simulink model "RLS_Self_maglev"  (R2023b)
settings: Solver=VariableStepAuto  StartTime=0.0  StopTime=5  RelTol=1e-3
undefined symbols (not defined in the file or in its folder): A_ob, B_ob, C_ob, D_ob, x1_eq0, x2_eq0
settings Model: Creator=Simone Garatti  LastModifiedBy=lollo
settings SolverCC: AlgebraicLoopSolver=TrustRegion
settings DataIOCC: ReturnWorkspaceOutputs=off
settings DebuggingCC: UnconnectedInputMsg=warning  UnconnectedOutputMsg=warning  UnconnectedLineMsg=warning  ArithmeticOperatorsInVariantConditions=warning
settings ModelReferenceCC: EnableRefExpFcnMdlSchedulingChecks=on
settings SFSimCC: CustomCodeUndefinedFunction=UseInterfaceOnly

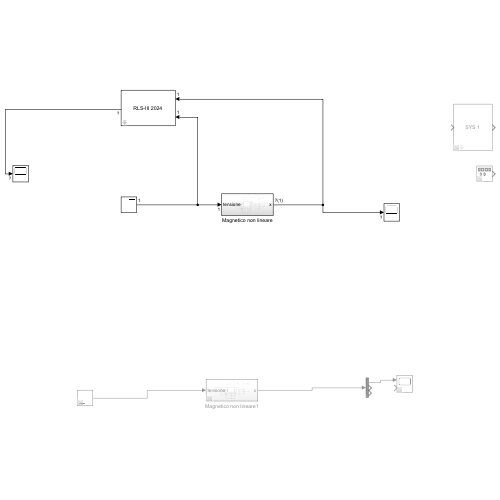
[thumbnail: Simulink's stored preview of the top-level diagram]
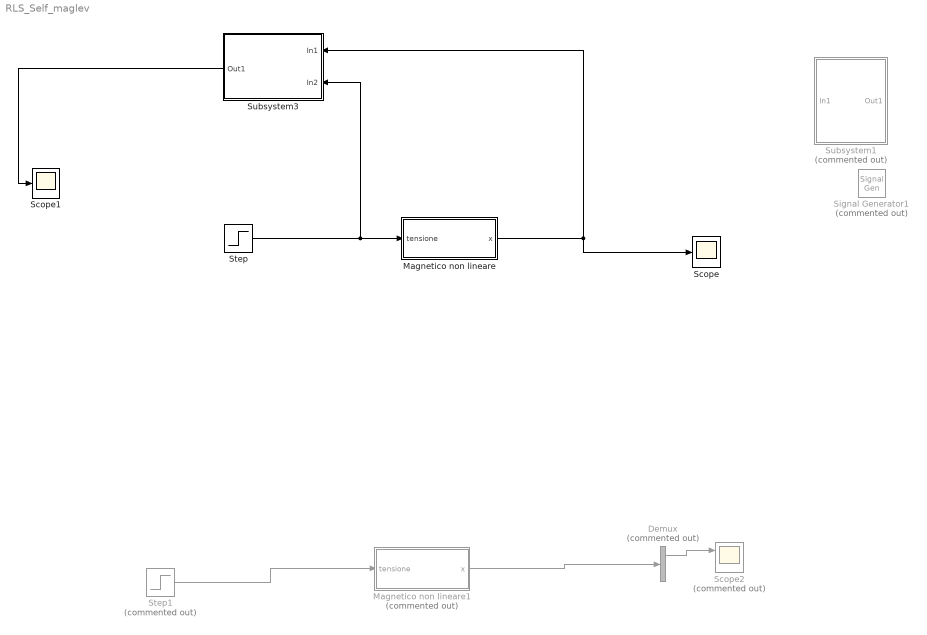
== system RLS_Self_maglev ==
  Demux : Demux  Commented=on  Outputs=3
  Magnetico non lineare : Subsystem
  Magnetico non lineare1 : Subsystem  Commented=on
  Scope : Scope
  Scope1 : Scope
  Scope2 : Scope  Commented=on  NumInputPorts=2
  Signal Generator1 : SignalGenerator  Commented=on  WaveForm=square  Frequency=0.01
  Step : Step  After=16  SampleTime=0
  Step1 : Step  Commented=on  After=20  SampleTime=0
  Subsystem1 : Subsystem  Commented=on  mask{yi=0, ui=0}
      mask prompts: yi "y(0)"; ui "u(0)"
      mask Display: disp('SYS 1')
  Subsystem3 : Subsystem  mask{th0=[2 3 2]', S0=eye(3)/100, ny=2, nu=0, d=1, mu=1}
      mask prompts: th0 "theta init"; S0 "S init"; d "u-y delay"; mu "forgetting factor"
      mask Display: disp('RLS-III 2024')
  wires:
  Step/1 -> Subsystem3/2(In2), Magnetico non lineare/1(tensione)
  Magnetico non lineare/1(x) -> Scope/1, Subsystem3/1(In1)
  Subsystem3/1(Out1) -> Scope1/1
  Step1/1 -> Magnetico non lineare1/1(tensione)
  Demux/1 -> Scope2/1
  Magnetico non lineare1/1(x) -> Demux/1

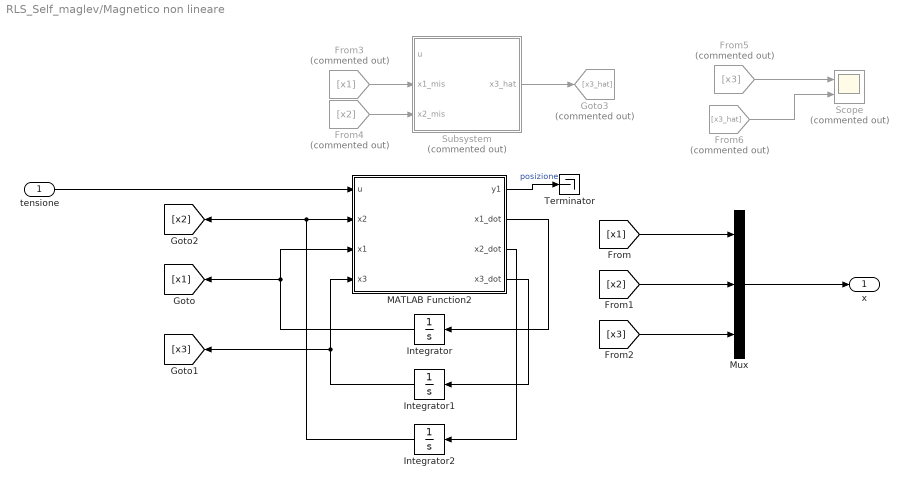
== system RLS_Self_maglev/Magnetico non lineare ==
  tensione : Inport
  From3 : From  Commented=on  GotoTag=x1
  From4 : From  Commented=on  GotoTag=x2
  From5 : From  Commented=on  GotoTag=x3
  From6 : From  Commented=on  GotoTag=x3_hat
  Goto3 : Goto  Commented=on  GotoTag=x3_hat
  Integrator : Integrator
  Integrator1 : Integrator
  Integrator2 : Integrator
  MATLAB Function2 : MATLAB Function  TreatAsAtomicUnit=on
  Mux : Mux  Inputs=3
  Scope : Scope  Commented=on  NumInputPorts=2
  Subsystem : Subsystem  Commented=on
  Terminator : Terminator
  x : Outport
  wires:
  tensione/1 -> MATLAB Function2/1(u)
  MATLAB Function2/2(x1_dot) -> Integrator/1
  Integrator/1 -> MATLAB Function2/3(x1), [x1]
  MATLAB Function2/4(x3_dot) -> Integrator1/1
  Integrator1/1 -> [x3], MATLAB Function2/4(x3)
  [x1] -> Mux/1
  [x2] -> Mux/2
  [x3] -> Mux/3
  Mux/1 -> x/1
  MATLAB Function2/3(x2_dot) -> Integrator2/1
  Integrator2/1 -> MATLAB Function2/2(x2), [x2]
  From3/1 -> Subsystem/2(x1_mis)
  From4/1 -> Subsystem/3(x2_mis)
  Subsystem/1(x3_hat) -> Goto3/1
  From6/1 -> Scope/2
  From5/1 -> Scope/1
  MATLAB Function2/1(y1) -> Terminator/1  "posizione"

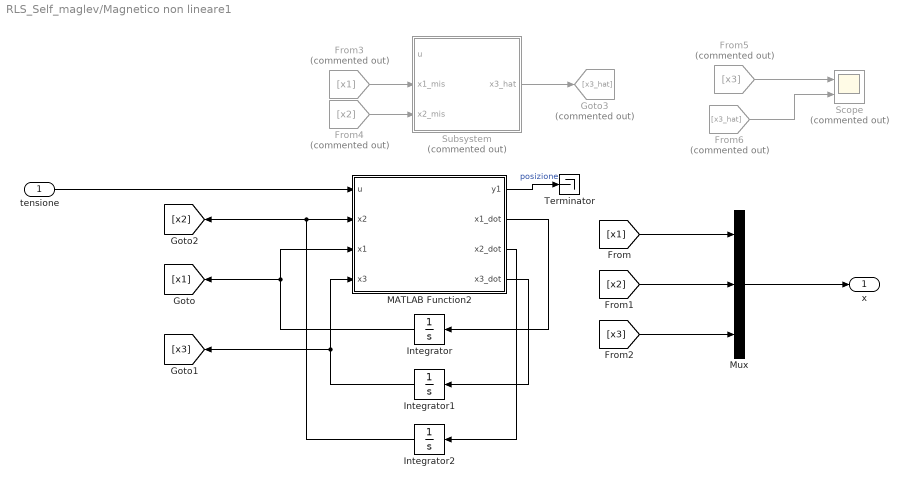
== system RLS_Self_maglev/Magnetico non lineare1 ==
  tensione : Inport
  From3 : From  Commented=on  GotoTag=x1
  From4 : From  Commented=on  GotoTag=x2
  From5 : From  Commented=on  GotoTag=x3
  From6 : From  Commented=on  GotoTag=x3_hat
  Goto3 : Goto  Commented=on  GotoTag=x3_hat
  Integrator : Integrator
  Integrator1 : Integrator
  Integrator2 : Integrator
  MATLAB Function2 : MATLAB Function  TreatAsAtomicUnit=on
  Mux : Mux  Inputs=3
  Scope : Scope  Commented=on  NumInputPorts=2
  Subsystem : Subsystem  Commented=on
  Terminator : Terminator
  x : Outport
  wires:
  tensione/1 -> MATLAB Function2/1(u)
  MATLAB Function2/2(x1_dot) -> Integrator/1
  Integrator/1 -> MATLAB Function2/3(x1), [x1]
  MATLAB Function2/4(x3_dot) -> Integrator1/1
  Integrator1/1 -> [x3], MATLAB Function2/4(x3)
  [x1] -> Mux/1
  [x2] -> Mux/2
  [x3] -> Mux/3
  Mux/1 -> x/1
  MATLAB Function2/3(x2_dot) -> Integrator2/1
  Integrator2/1 -> MATLAB Function2/2(x2), [x2]
  From3/1 -> Subsystem/2(x1_mis)
  From4/1 -> Subsystem/3(x2_mis)
  Subsystem/1(x3_hat) -> Goto3/1
  From6/1 -> Scope/2
  From5/1 -> Scope/1
  MATLAB Function2/1(y1) -> Terminator/1  "posizione"

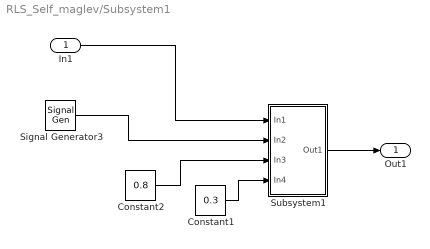
== system RLS_Self_maglev/Subsystem1 ==
  In1 : Inport
  Constant1 : Constant  Value=0.3
  Constant2 : Constant  Value=0.8
  Signal Generator3 : SignalGenerator  WaveForm=random  Amplitude=0.0  Frequency=0.01
  Subsystem1 : Subsystem  mask{y0=yi, u0=ui}
      mask prompts: y0 "y(0)"; u0 "u(0)"
      mask Display: disp('SYS')
  Out1 : Outport  VectorParamsAs1DForOutWhenUnconnected=off
  wires:
  Signal Generator3/1 -> Subsystem1/2(In2)
  Subsystem1/1(Out1) -> Out1/1
  Constant1/1 -> Subsystem1/4(In4)
  In1/1 -> Subsystem1/1(In1)
  Constant2/1 -> Subsystem1/3(In3)

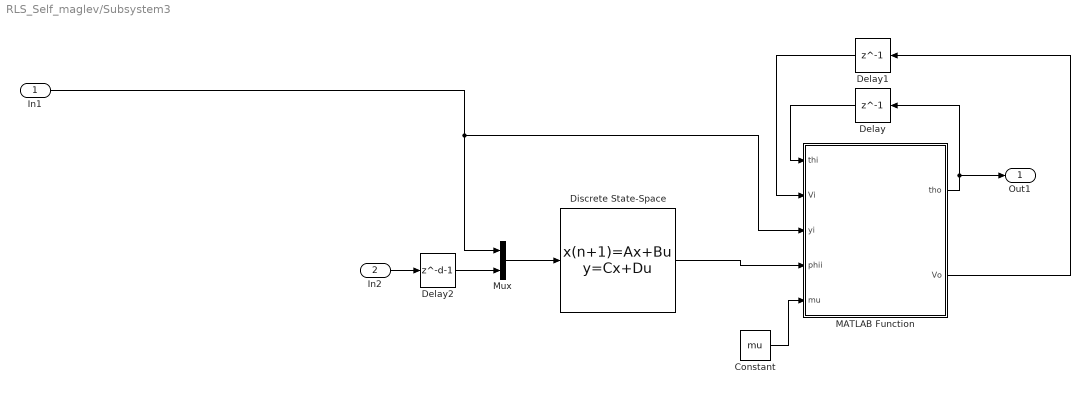
== system RLS_Self_maglev/Subsystem3 ==
  In1 : Inport
  In2 : Inport  Port=2
  Constant : Constant  Value=mu
  Delay : Delay  DelayLength=1  InitialCondition=th0
  Delay1 : Delay  DelayLength=1  InitialCondition=inv(S0)
  Delay2 : Delay  DelayLength=d-1  InitialCondition=0
  Discrete State-Space : DiscreteStateSpace  A=[ diag(ones(ny-1,1),-1) zeros(ny,nu+1); zeros(nu+1,ny) diag(ones(nu,1),-1) ]  B=[[1 0]; zeros(ny-1,2); [0 1]; zeros(nu,2)]  C=eye(ny+nu+1)  D=zeros(ny+nu+1,2)  SampleTime=-1
  MATLAB Function : MATLAB Function  TreatAsAtomicUnit=on
  Mux : Mux  Inputs=2
  Out1 : Outport  VectorParamsAs1DForOutWhenUnconnected=off
  wires:
  MATLAB Function/1(tho) -> Delay/1, Out1/1
  Delay/1 -> MATLAB Function/1(thi)
  MATLAB Function/2(Vo) -> Delay1/1
  Delay1/1 -> MATLAB Function/2(Vi)
  In1/1 -> Mux/1, MATLAB Function/3(yi)
  In2/1 -> Delay2/1
  Delay2/1 -> Mux/2
  Mux/1 -> Discrete State-Space/1
  Discrete State-Space/1 -> MATLAB Function/4(phii)
  Constant/1 -> MATLAB Function/5(mu)

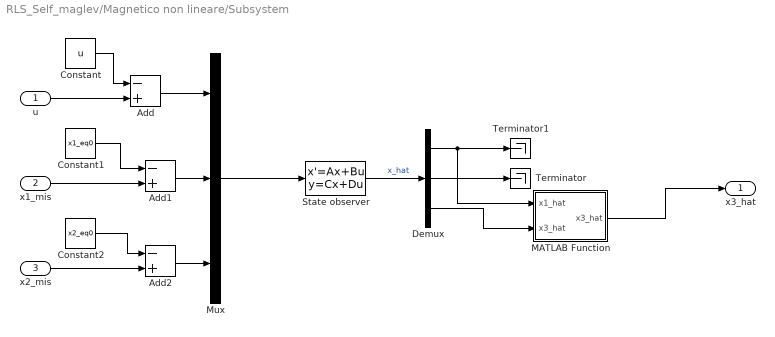
== system RLS_Self_maglev/Magnetico non lineare/Subsystem ==
  u : Inport
  x1_mis : Inport  Port=2
  x2_mis : Inport  Port=3
  Add : Sum  Inputs=-+
  Add1 : Sum  Inputs=-+
  Add2 : Sum  Inputs=-+
  Constant : Constant  Value=u
  Constant1 : Constant  Value=x1_eq0
  Constant2 : Constant  Value=x2_eq0
  Demux : Demux  Outputs=3
  MATLAB Function : MATLAB Function  TreatAsAtomicUnit=on
  Mux : Mux  Inputs=3
  State observer : StateSpace  A=A_ob  B=B_ob  C=C_ob  D=D_ob  InitialCondition=[0;0;0]  ParameterTunability=Unconstrained
  Terminator : Terminator
  Terminator1 : Terminator
  x3_hat : Outport
  wires:
  x1_mis/1 -> Add1/2
  u/1 -> Add/2
  Mux/1 -> State observer/1
  State observer/1 -> Demux/1  "x_hat"
  Demux/1 -> MATLAB Function/1(x1_hat), Terminator1/1
  Demux/2 -> Terminator/1
  Constant/1 -> Add/1
  Constant1/1 -> Add1/1
  Constant2/1 -> Add2/1
  x2_mis/1 -> Add2/2
  Add/1 -> Mux/1
  Add1/1 -> Mux/2
  Add2/1 -> Mux/3
  MATLAB Function/1(x3_hat) -> x3_hat/1
  Demux/3 -> MATLAB Function/2("x3_hat ")

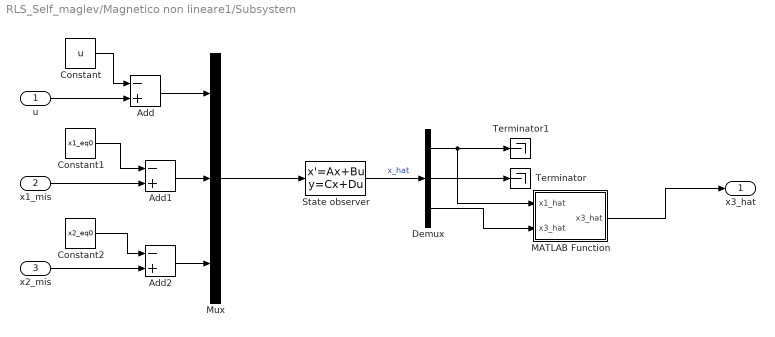
== system RLS_Self_maglev/Magnetico non lineare1/Subsystem ==
  u : Inport
  x1_mis : Inport  Port=2
  x2_mis : Inport  Port=3
  Add : Sum  Inputs=-+
  Add1 : Sum  Inputs=-+
  Add2 : Sum  Inputs=-+
  Constant : Constant  Value=u
  Constant1 : Constant  Value=x1_eq0
  Constant2 : Constant  Value=x2_eq0
  Demux : Demux  Outputs=3
  MATLAB Function : MATLAB Function  TreatAsAtomicUnit=on
  Mux : Mux  Inputs=3
  State observer : StateSpace  A=A_ob  B=B_ob  C=C_ob  D=D_ob  InitialCondition=[0;0;0]  ParameterTunability=Unconstrained
  Terminator : Terminator
  Terminator1 : Terminator
  x3_hat : Outport
  wires:
  x1_mis/1 -> Add1/2
  u/1 -> Add/2
  Mux/1 -> State observer/1
  State observer/1 -> Demux/1  "x_hat"
  Demux/1 -> MATLAB Function/1(x1_hat), Terminator1/1
  Demux/2 -> Terminator/1
  Constant/1 -> Add/1
  Constant1/1 -> Add1/1
  Constant2/1 -> Add2/1
  x2_mis/1 -> Add2/2
  Add/1 -> Mux/1
  Add1/1 -> Mux/2
  Add2/1 -> Mux/3
  MATLAB Function/1(x3_hat) -> x3_hat/1
  Demux/3 -> MATLAB Function/2("x3_hat ")

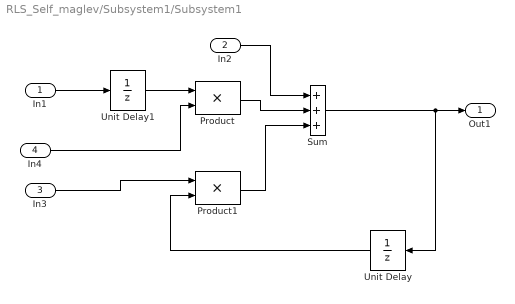
== system RLS_Self_maglev/Subsystem1/Subsystem1 ==
  In1 : Inport
  In2 : Inport  Port=2
  In3 : Inport  Port=3
  In4 : Inport  Port=4
  Product : Product  SaturateOnIntegerOverflow=on  OutDataTypeStr=Inherit: Same as first input
  Product1 : Product  SaturateOnIntegerOverflow=on  OutDataTypeStr=Inherit: Same as first input
  Sum : Sum  Inputs=+++  SaturateOnIntegerOverflow=on
  Unit Delay : UnitDelay  InitialCondition=y0  HasFrameUpgradeWarning=on
  Unit Delay1 : UnitDelay  InitialCondition=u0  HasFrameUpgradeWarning=on
  Out1 : Outport  VectorParamsAs1DForOutWhenUnconnected=off
  wires:
  In2/1 -> Sum/1
  Product/1 -> Sum/2
  In3/1 -> Product1/1
  In4/1 -> Product/2
  Product1/1 -> Sum/3
  Unit Delay/1 -> Product1/2
  Sum/1 -> Unit Delay/1, Out1/1
  Unit Delay1/1 -> Product/1
  In1/1 -> Unit Delay1/1

== matlab function RLS_Self_maglev/Subsystem3/MATLAB Function ==
  data: thi input; tho output; Vi input; yi input; phii input; Vo output; mu input
function [tho,Vo] = updaterule(thi,Vi,yi,phii,mu)

Vo = Vi/mu - (Vi*phii*phii'*Vi)/(mu+phii'*Vi*phii)/mu;
tho = thi + Vo*phii*(yi-phii'*thi);

== matlab function RLS_Self_maglev/Magnetico non lineare1/MATLAB Function2 ==
  data: u input; y1 output; x2 input; x1_dot output; x2_dot output; x1 input; x3 input; x3_dot output
function [y1,x1_dot, x2_dot, x3_dot] = fcn(u, x2, x1, x3)
    m = 0.0657;
    g = 9.81;
    k_mag = 2.4405e-05;
    Rtot = 9.7585;
    Lc = 0.3708;
    y0 = 0.012;
    
    x2_dot = 1/Lc*(-Rtot*x2 + u);

    x1_dot = x3;
    if x1 < y0
        x3_dot = (k_mag/m)*(x2/(y0-x1))^2 - g;
    else
        x1 = 0.012;
        x3_dot = 0;
        x3 = 0;
    end

    
    % condizioni
    if x1 <=0 && x3_dot < 0
        x1 = 0;
        x3 = 0;
        x3_dot = 0;
    end
y1 = x1;

== matlab function RLS_Self_maglev/Magnetico non lineare/Subsystem/MATLAB Function ==
  data: x1_hat input; x3_hat output; x3_hat input
function x3_hat = fcn(x1_hat, x3_hat)

if x1_hat<=0 && x3_hat<=0
    x3_hat=0;
end

== matlab function RLS_Self_maglev/Magnetico non lineare/MATLAB Function2 ==
  data: u input; y1 output; x2 input; x1_dot output; x2_dot output; x1 input; x3 input; x3_dot output
function [y1,x1_dot, x2_dot, x3_dot] = fcn(u, x2, x1, x3)
    m = 0.0657;
    g = 9.81;
    k_mag = 2.4405e-05;
    Rtot = 9.7585;
    Lc = 0.3708;
    y0 = 0.012;
    
    x2_dot = 1/Lc*(-Rtot*x2 + u);

    x1_dot = x3;
    if x1 < y0
        x3_dot = (k_mag/m)*(x2/(y0-x1))^2 - g;
    else
        x1 = 0.012;
        x3_dot = 0;
        x3 = 0;
    end

    
    % condizioni
    if x1 <=0 && x3_dot < 0
        x1 = 0;
        x3 = 0;
        x3_dot = 0;
    end
y1 = x1;

== matlab function RLS_Self_maglev/Magnetico non lineare1/Subsystem/MATLAB Function ==
  data: x1_hat input; x3_hat output; x3_hat input
function x3_hat = fcn(x1_hat, x3_hat)

if x1_hat<=0 && x3_hat<=0
    x3_hat=0;
end
